simulink library "drv_ld_time_v0"  (R2016a)
settings: Solver=ode45  StartTime=0.0  StopTime=10.0  RelTol=1e-3
undefined symbols (not defined in the file): DiscIntNeverNeededParam, sMP
libraries: simulink x5
settings Model: Creator=LAUEREL  LastModifiedBy=UWLELKE
settings DataIOCC: LimitDataPoints=on  SaveFormat=Array
settings OptimizationCC: ExpressionDepthLimit=2147483647
settings DebuggingCC: UnderspecifiedInitializationDetection=Classic  MergeDetectMultiDrivingBlocksExec=none  SolverPrmCheckMsg=warning  StateNameClashWarn=warning
settings HardwareCC: ProdBitPerPointer=32  ProdLargestAtomicFloat=None  ProdIntDivRoundTo=Undefined  ProdEndianess=Unspecified  ProdWordSize=32  ProdHWDeviceType=32-bit Generic
settings ModelReferenceCC: PropagateSignalLabelsOutOfModel=off

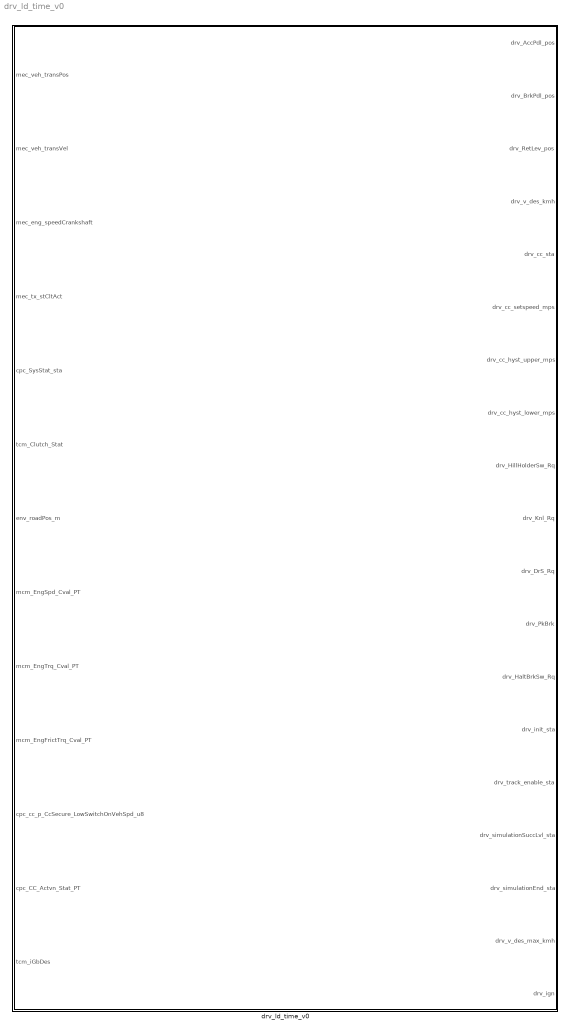
== system drv_ld_time_v0 ==
  drv_ld_time_v0 : Subsystem  TreatAsAtomicUnit=on  mask(DrivereDrive){aeroCdA_m2=sMP.human.drv.aeroCdA_m2, aeroRhoAirDensity_kgpm3=sMP.human.drv.aeroRhoAirDensity_kgpm3, coefReRollgVeh=sMP.human.drv.coefReRollgVeh, aGrv=sMP.human.drv.aGrv, Vehicle_Mass=sMP.human.drv.mass_gcw_kg, rdyn=sMP.human.drv.rdyn, CYC=sMP.bdry.env.CYC, gearration=sMP.human.drv.gearration, Ki_Accln=sMP.human.drv.Ki_Accln, Ki_breaking=sMP.human.drv.Ki_breaking, Veh_Speed_Breaking=sMP.human.drv.Veh_Speed_Breaking, veh_speed_accln=sMP.human.drv.veh_speed_accln, Kp_grad_Accln=sMP.human.drv.Kp_grad_Accln, Kp_grad_breaking=sMP.human.drv.Kp_grad_breaking, Grad_breaking=sMP.human.drv.Grad_breaking, Grad_Accln=sMP.human.drv.Grad_Accln, Mmax_motor=sMP.human.drv.Mmax_motor, vehPara_AccPdlCurve=sMP.human.drv.vehPara.AccPdlCurve, vehPara_BrkPdlCurve=sMP.human.drv.vehPara.BrkPdlCurve, Corr_const=sMP.human.drv.Corr_const, Kp_corr=sMP.human.drv.Kp_corr, Kp_acc_const=sMP.human.drv.Kp_acc_const, Kp_brk_const=sMP.human.drv.Kp_brk_const, corr_tuning=sMP.human.drv.corr_tuning, Ki_acc_const=sMP.human.drv.Ki_acc_const, Ki_brk_const=sMP.human.drv.Ki_brk_const, Kp_v=sMP.human.drv.Kp_v, Kp_acc=sMP.human.drv.Kp_acc, Kp_brk=sMP.human.drv.Kp_brk, Ki=sMP.human.drv.Ki, Ki_gain=sMP.human.drv.Ki_gain, refMass=sMP.human.drv.refMass}
      mask prompts: Vehicle_Mass "mass_gcw_kg"; CYC "cycleparameter"; gearration "gear ratio"
      mask help:
      | Set the struct variables for driver parameters (veh) and route data (cyc).
      |
      | eDrive Driver
      | This driver is able to drive time based cycles.

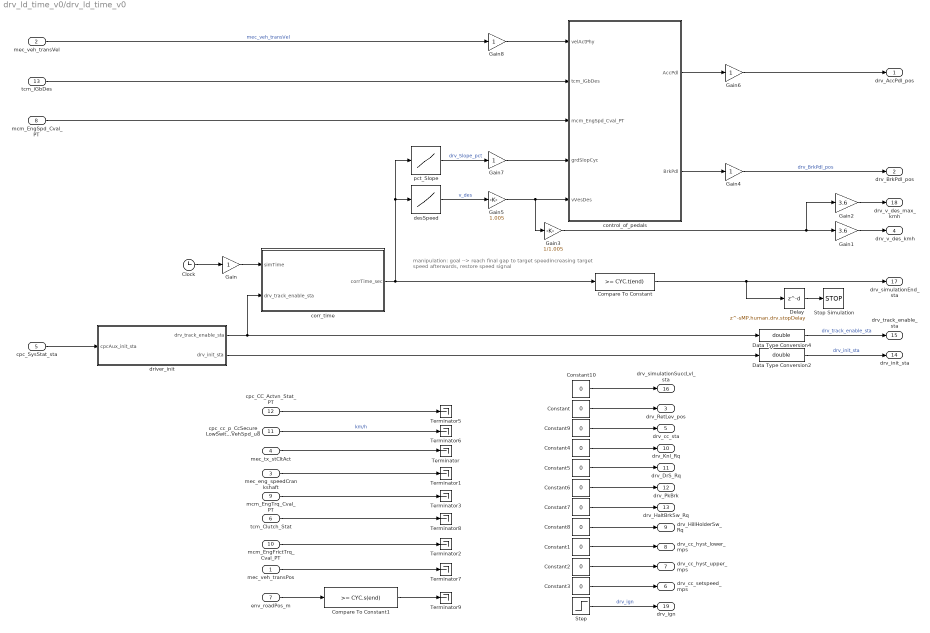
== system drv_ld_time_v0/drv_ld_time_v0 ==
  note: manipulation:
      | goal --> reach final gap to target speedincreasing target speed
      | afterwards, restore speed signal
  mec_veh_transPos : Inport
  mec_veh_transVel : Inport  Port=2
  mec_eng_speedCrankshaft : Inport  Port=3
  mec_tx_stCltAct : Inport  Port=4
  cpc_SysStat_sta : Inport  Port=5
  tcm_Clutch_Stat : Inport  Port=6
  env_roadPos_m : Inport  Port=7
  mcm_EngSpd_Cval_PT : Inport  Port=8
  mcm_EngTrq_Cval_PT : Inport  Port=9
  mcm_EngFrictTrq_Cval_PT : Inport  Port=10
  cpc_cc_p_CcSecure_LowSwitchOnVehSpd_u8 : Inport  Port=11
  cpc_CC_Actvn_Stat_PT : Inport  Port=12
  tcm_iGbDes : Inport  Port=13
  Clock : Clock
  Compare To Constant : simulink/Logic and Bit Operations/Compare To Constant  relop=>=  const=CYC.t(end)  OutDataTypeStr=boolean
  Compare To Constant1 : simulink/Logic and Bit Operations/Compare To Constant  relop=>=  const=CYC.s(end)  OutDataTypeStr=boolean
  Constant{,1..10} (11 alike) : Constant  Value=0
  Data Type Conversion2 : DataTypeConversion  OutDataTypeStr=double
  Data Type Conversion4 : DataTypeConversion  OutDataTypeStr=double
  Delay : Delay  DelayLength=sMP.human.drv.stopDelay  InitialCondition=0
  Gain : Gain  SampleTime=K
      mask init:
      | K = str2num(get_param(bdroot,'FixedStep'));
  Gain1 : Gain  Gain=3.6
  Gain2 : Gain  Gain=3.6
  Gain3 : Gain  Gain=1/1.005
      settings: AttributesFormatString=%<Gain>
  Gain{4,6..8} (4 alike) : Gain
  Gain5 : Gain  Gain=1.005
      settings: AttributesFormatString=%<Gain>
  Step : Step  Time=0.1  SampleTime=0
      settings: AttributesFormatString=%<Before> >> %<After> after %<Time>s
  Stop Simulation : Stop
  Terminator{,1..3,5..9} (9 alike) : Terminator
  control_of_pedals : Subsystem
  corr_time : Subsystem
  desSpeed : Lookup  InputValues=CYC.t  Table=CYC.v
  driver_init : Subsystem
  pct_Slope : Lookup  InputValues=CYC.t  Table=CYC.grade
  drv_AccPdl_pos : Outport
  drv_BrkPdl_pos : Outport  Port=2
  drv_RetLev_pos : Outport  Port=3
  drv_v_des_kmh : Outport  Port=4
  drv_cc_sta : Outport  Port=5
  drv_cc_setspeed_mps : Outport  Port=6
  drv_cc_hyst_upper_mps : Outport  Port=7
  drv_cc_hyst_lower_mps : Outport  Port=8
  drv_HillHolderSw_Rq : Outport  Port=9
  drv_Knl_Rq : Outport  Port=10
  drv_DrS_Rq : Outport  Port=11
  drv_PkBrk : Outport  Port=12
  drv_HaltBrkSw_Rq : Outport  Port=13
  drv_init_sta : Outport  Port=14
  drv_track_enable_sta : Outport  Port=15
  drv_simulationSuccLvl_sta : Outport  Port=16
  drv_simulationEnd_sta : Outport  Port=17
  drv_v_des_max_kmh : Outport  Port=18
  drv_ign : Outport  Port=19
  wires:
  mcm_EngFrictTrq_Cval_PT/1 -> Terminator2/1
  Constant10/1 -> drv_simulationSuccLvl_sta/1
  Delay/1 -> Stop Simulation/1
  Step/1 -> drv_ign/1  "drv_ign"
  tcm_iGbDes/1 -> control_of_pedals/2(tcm_iGbDes)
  mec_veh_transPos/1 -> Terminator7/1
  corr_time/1(corrTime_sec) -> pct_Slope/1, desSpeed/1, Compare To Constant/1
  Clock/1 -> Gain/1
  desSpeed/1 -> Gain5/1  "v_des"
  Constant/1 -> drv_RetLev_pos/1
  Constant9/1 -> drv_cc_sta/1
  Constant5/1 -> drv_DrS_Rq/1
  Constant6/1 -> drv_PkBrk/1
  Constant7/1 -> drv_HaltBrkSw_Rq/1
  Constant8/1 -> drv_HillHolderSw_Rq/1
  Constant4/1 -> drv_Knl_Rq/1
  Constant3/1 -> drv_cc_setspeed_mps/1
  Constant2/1 -> drv_cc_hyst_upper_mps/1
  Constant1/1 -> drv_cc_hyst_lower_mps/1
  tcm_Clutch_Stat/1 -> Terminator8/1
  mcm_EngTrq_Cval_PT/1 -> Terminator3/1
  mcm_EngSpd_Cval_PT/1 -> control_of_pedals/3(mcm_EngSpd_Cval_PT)
  mec_eng_speedCrankshaft/1 -> Terminator1/1
  mec_tx_stCltAct/1 -> Terminator/1
  cpc_cc_p_CcSecure_LowSwitchOnVehSpd_u8/1 -> Terminator6/1  "km/h"
  cpc_CC_Actvn_Stat_PT/1 -> Terminator5/1
  mec_veh_transVel/1 -> Gain8/1  "mec_veh_transVel"
  pct_Slope/1 -> Gain7/1  "drv_Slope_pct"
  cpc_SysStat_sta/1 -> driver_init/1(cpcAux_init_sta)
  driver_init/1(drv_track_enable_sta) -> corr_time/2(drv_track_enable_sta), Data Type Conversion4/1
  env_roadPos_m/1 -> Compare To Constant1/1
  Data Type Conversion4/1 -> drv_track_enable_sta/1  "drv_track_enable_sta"
  Data Type Conversion2/1 -> drv_init_sta/1  "drv_init_sta"
  driver_init/2(drv_init_sta) -> Data Type Conversion2/1
  Gain1/1 -> drv_v_des_kmh/1
  Gain2/1 -> drv_v_des_max_kmh/1
  Gain/1 -> corr_time/1(simTime)
  Compare To Constant/1 -> drv_simulationEnd_sta/1, Delay/1
  Compare To Constant1/1 -> Terminator9/1
  control_of_pedals/1(AccPdl) -> Gain6/1
  Gain4/1 -> drv_BrkPdl_pos/1  "drv_BrkPdl_pos"
  control_of_pedals/2(BrkPdl) -> Gain4/1
  Gain6/1 -> drv_AccPdl_pos/1
  Gain7/1 -> control_of_pedals/4(grdSlopCyc)
  Gain8/1 -> control_of_pedals/1(velActPhy)
  Gain3/1 -> Gain2/1, Gain1/1
  Gain5/1 -> Gain3/1, control_of_pedals/5(vVesDes)

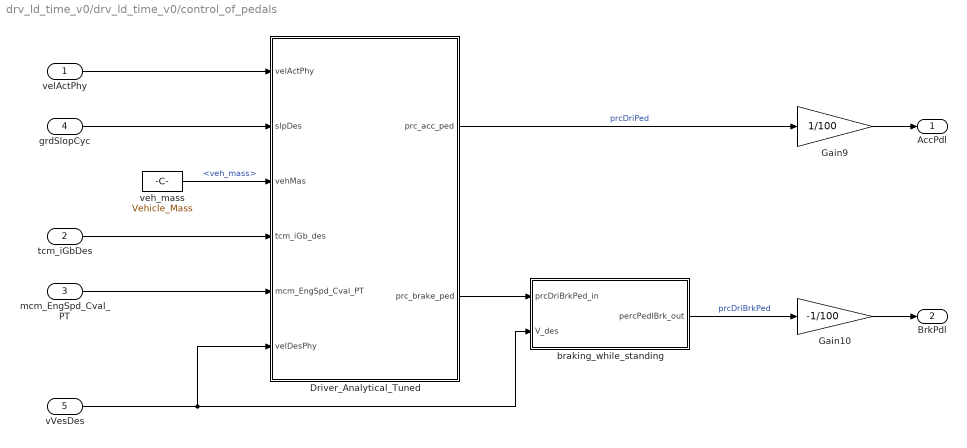
== system drv_ld_time_v0/drv_ld_time_v0/control_of_pedals ==
  velActPhy : Inport
  tcm_iGbDes : Inport  Port=2
  mcm_EngSpd_Cval_PT : Inport  Port=3
  grdSlopCyc : Inport  Port=4
  vVesDes : Inport  Port=5
  Driver_Analytical_Tuned : Subsystem
  Gain10 : Gain  Gain=-1/100
  Gain9 : Gain  Gain=1/100
  braking_while_standing : Subsystem
  veh_mass : Constant  Value=Vehicle_Mass
  AccPdl : Outport
  BrkPdl : Outport  Port=2
  wires:
  mcm_EngSpd_Cval_PT/1 -> Driver_Analytical_Tuned/5(mcm_EngSpd_Cval_PT)
  Driver_Analytical_Tuned/2(prc_brake_ped) -> braking_while_standing/1(prcDriBrkPed_in)
  braking_while_standing/1(percPedlBrk_out) -> Gain10/1  "prcDriBrkPed"
  tcm_iGbDes/1 -> Driver_Analytical_Tuned/4(tcm_iGb_des)
  veh_mass/1 -> Driver_Analytical_Tuned/3(vehMas)  "<veh_mass>"
  velActPhy/1 -> Driver_Analytical_Tuned/1(velActPhy)
  grdSlopCyc/1 -> Driver_Analytical_Tuned/2(slpDes)
  vVesDes/1 -> Driver_Analytical_Tuned/6(velDesPhy), braking_while_standing/2(V_des)
  Driver_Analytical_Tuned/1(prc_acc_ped) -> Gain9/1  "prcDriPed"
  Gain9/1 -> AccPdl/1
  Gain10/1 -> BrkPdl/1

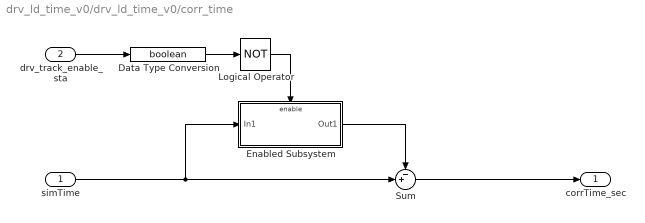
== system drv_ld_time_v0/drv_ld_time_v0/corr_time ==
  simTime : Inport
  drv_track_enable_sta : Inport  Port=2
  Data Type Conversion : DataTypeConversion  OutDataTypeStr=boolean
  Enabled Subsystem : Subsystem  TreatAsAtomicUnit=on
  Logical Operator : Logic  Operator=NOT  AllPortsSameDT=off  OutDataTypeStr=boolean
  Sum : Sum  Inputs=-+|
  corrTime_sec : Outport
  wires:
  Data Type Conversion/1 -> Logical Operator/1
  Sum/1 -> corrTime_sec/1
  Enabled Subsystem/1(Out1) -> Sum/1
  Logical Operator/1 -> Enabled Subsystem/Enable
  drv_track_enable_sta/1 -> Data Type Conversion/1
  simTime/1 -> Sum/2, Enabled Subsystem/1(In1)

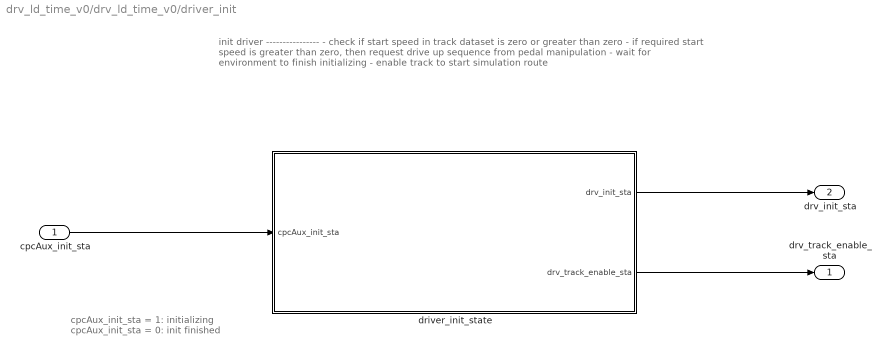
== system drv_ld_time_v0/drv_ld_time_v0/driver_init ==
  note: init driver
      | ----------------
      | - check if start speed in track dataset is zero or greater than zero
      | - if required start speed is greater than zero, then request drive up sequence from pedal manipulation
      | - wait for environment to finish initializing
      | - enable track to start simulation route
  note: cpcAux_init_sta = 1: initializing
      | cpcAux_init_sta = 0: init finished
  cpcAux_init_sta : Inport
  driver_init_state : Stateflow chart  TreatAsAtomicUnit=on
  drv_track_enable_sta : Outport
  drv_init_sta : Outport  Port=2
  wires:
  driver_init_state/1(drv_init_sta) -> drv_init_sta/1
  driver_init_state/2(drv_track_enable_sta) -> drv_track_enable_sta/1
  cpcAux_init_sta/1 -> driver_init_state/1(cpcAux_init_sta)

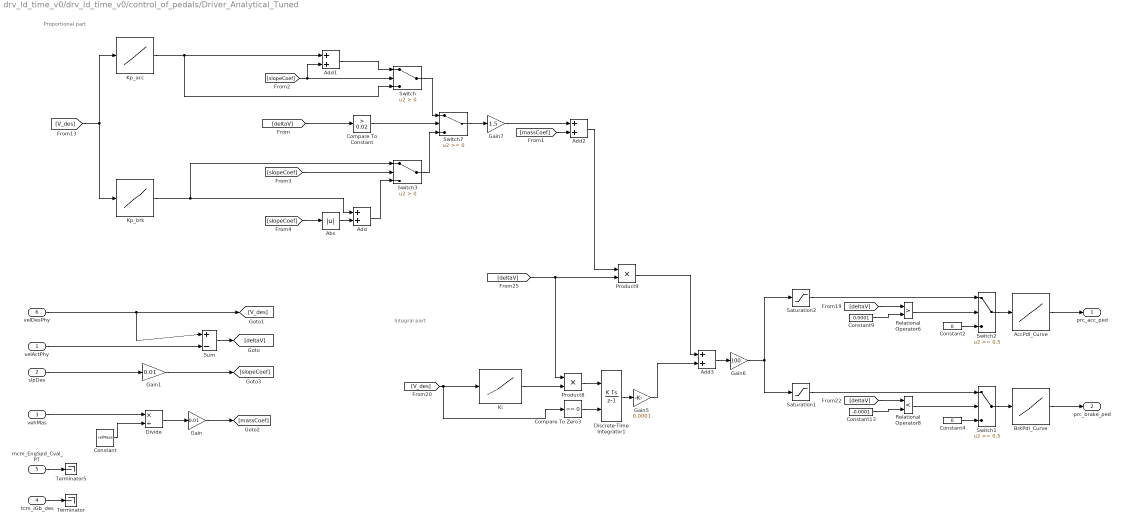
== system drv_ld_time_v0/drv_ld_time_v0/control_of_pedals/Driver_Analytical_Tuned ==
  note: Integral part
  note: Proportional part
  velActPhy : Inport
  slpDes : Inport  Port=2
  vehMas : Inport  Port=3
  tcm_iGb_des : Inport  Port=4
  mcm_EngSpd_Cval_PT : Inport  Port=5
  velDesPhy : Inport  Port=6
  Abs : Abs
  AccPdl_Curve : Lookup_n-D  NumberOfTableDimensions=1  BreakpointsForDimension1=vehPara_AccPdlCurve(:,1)  Table=vehPara_AccPdlCurve(:,2)  InternalRulePriority=Speed  RndMeth=Simplest  InputSameDT=on
  Add{,1..3} (4 alike) : Sum
  BrkPdl_Curve : Lookup_n-D  NumberOfTableDimensions=1  BreakpointsForDimension1=vehPara_BrkPdlCurve(:,1)  Table=vehPara_BrkPdlCurve(:,2)  InternalRulePriority=Speed  RndMeth=Simplest  InputSameDT=on
  Compare To Constant : simulink/Logic and Bit Operations/Compare To Constant  relop=>  const=0.02  OutDataTypeStr=boolean
  Compare To Zero3 : simulink/Logic and Bit Operations/Compare To Zero  relop===  OutDataTypeStr=boolean
  Constant : Constant  Value=refMass
      settings: AttributesFormatString=%<Value>
  Constant13 : Constant  Value=-0.0001
  Constant2 : Constant  Value=0
  Constant4 : Constant  Value=0
  Constant9 : Constant  Value=0.0001
  Discrete-Time Integrator1 : DiscreteIntegrator  ExternalReset=level  SampleTime=-1  LimitOutput=on  UpperSaturationLimit=7500  LowerSaturationLimit=-7500  ICPrevOutput=DiscIntNeverNeededParam  ICPrevScaledInput=DiscIntNeverNeededParam
  Divide : Product  Inputs=*/
  Gain : Gain  Gain=0.01
      settings: AttributesFormatString=%<Gain>
  Gain1 : Gain  Gain=0.01
  Gain5 : Gain  Gain=0.0001
      settings: AttributesFormatString=%<Gain>
  Gain6 : Gain  Gain=100
  Gain7 : Gain  Gain=1.5
      settings: AttributesFormatString=%<Gain>
  Ki : Lookup_n-D  NumberOfTableDimensions=1  BreakpointsForDimension1=[0,10,20,30,40,50,60,70,80]  BreakpointsForDimension2=Veh_Speed_Breaking  Table=[0.01,0.015,0.02,0.0225,0.03,0.035,0.04,0.045,0.05]  RndMeth=Simplest  InputSameDT=on
  Kp_acc : Lookup_n-D  NumberOfTableDimensions=1  BreakpointsForDimension1=Kp_acc(2,:)  BreakpointsForDimension2=Veh_Speed_Breaking  Table=Kp_acc(1,:)  RndMeth=Simplest  InputSameDT=on
  Kp_brk : Lookup_n-D  NumberOfTableDimensions=1  BreakpointsForDimension1=[0,10,20,30,40,50,60,70,80,90,100]  BreakpointsForDimension2=Veh_Speed_Breaking  Table=[1,1.25,1.25,1.5,1.5,1.5,1.7,1.8,1.8,1.8,2]*0.1  RndMeth=Simplest  InputSameDT=on
  Product8 : Product
  Product9 : Product
  Relational Operator6 : RelationalOperator  Operator=>  OutDataTypeStr=uint(8)
  Relational Operator8 : RelationalOperator  Operator=<  OutDataTypeStr=uint(8)
  Saturation1 : Saturate  UpperLimit=0  LowerLimit=-100
      settings: AttributesFormatString=%<UpperLimit>\n%<LowerLimit>
  Saturation2 : Saturate  UpperLimit=100  LowerLimit=0
      settings: AttributesFormatString=%<UpperLimit>\n%<LowerLimit>
  Sum : Sum  Inputs=|+-
  Switch : Switch  Criteria=u2 > Threshold
  Switch1 : Switch  Threshold=0.5
  Switch2 : Switch  Threshold=0.5
  Switch3 : Switch  Criteria=u2 > Threshold
  Switch7 : Switch
  Terminator : Terminator
  Terminator5 : Terminator
  prc_acc_ped : Outport
  prc_brake_ped : Outport  Port=2
  wires:
  Gain7/1 -> Add2/1
  Gain/1 -> [massCoef]
  Gain1/1 -> [slopeCoef]
  [massCoef] -> Add2/2
  Divide/1 -> Gain/1
  Add2/1 -> Product9/1
  Switch7/1 -> Gain7/1
  [deltaV] -> Product8/1, Product9/2
  Add1/1 -> Switch/1
  Product9/1 -> Add3/1
  Kp_brk/1 -> Switch3/1, Add/1
  Switch3/1 -> Switch7/3
  [slopeCoef] -> Switch3/2
  Kp_acc/1 -> Switch/3, Add1/1
  Switch/1 -> Switch7/1
  Constant/1 -> Divide/2
  Sum/1 -> [deltaV]
  Compare To Constant/1 -> Switch7/2
  Discrete-Time Integrator1/1 -> Gain5/1
  Compare To Zero3/1 -> Discrete-Time Integrator1/2
  [V_des] -> Ki/1, Compare To Zero3/1
  [deltaV] -> Compare To Constant/1
  [V_des] -> Kp_acc/1, Kp_brk/1
  Gain6/1 -> Saturation1/1, Saturation2/1
  Add3/1 -> Gain6/1
  Product8/1 -> Discrete-Time Integrator1/1
  Relational Operator8/1 -> Switch1/2
  [deltaV] -> Relational Operator8/1
  Constant13/1 -> Relational Operator8/2
  Relational Operator6/1 -> Switch2/2
  [deltaV] -> Relational Operator6/1
  Constant9/1 -> Relational Operator6/2
  mcm_EngSpd_Cval_PT/1 -> Terminator5/1
  velActPhy/1 -> Sum/2
  AccPdl_Curve/1 -> prc_acc_ped/1
  BrkPdl_Curve/1 -> prc_brake_ped/1
  tcm_iGb_des/1 -> Terminator/1
  velDesPhy/1 -> [V_des], Sum/1
  slpDes/1 -> Gain1/1
  vehMas/1 -> Divide/1
  Saturation2/1 -> Switch2/1
  Saturation1/1 -> Switch1/1
  Switch2/1 -> AccPdl_Curve/1
  Switch1/1 -> BrkPdl_Curve/1
  Constant4/1 -> Switch1/3
  Constant2/1 -> Switch2/3
  [slopeCoef] -> Switch/2, Add1/2
  [slopeCoef] -> Abs/1
  Abs/1 -> Add/2
  Add/1 -> Switch3/3
  Gain5/1 -> Add3/2
  Ki/1 -> Product8/2

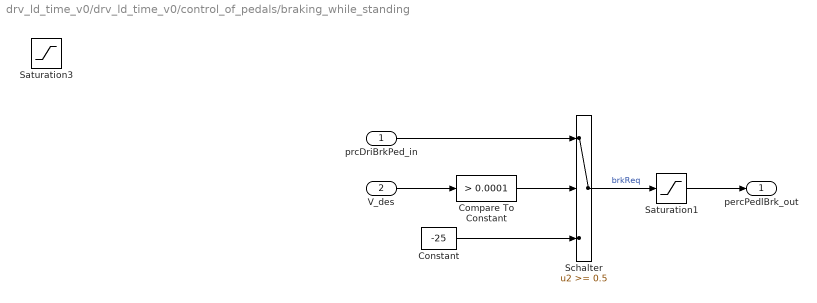
== system drv_ld_time_v0/drv_ld_time_v0/control_of_pedals/braking_while_standing ==
  prcDriBrkPed_in : Inport
  V_des : Inport  Port=2
  Compare To Constant : simulink/Logic and Bit Operations/Compare To Constant  relop=>  const=0.0001  OutDataTypeStr=boolean
  Constant : Constant  Value=-25
      settings: AttributesFormatString=%<Value>
  Saturation1 : Saturate  UpperLimit=0  LowerLimit=-100
      settings: AttributesFormatString=%<UpperLimit>\n%<LowerLimit>
  Saturation3 : Saturate  UpperLimit=0  LowerLimit=-100
      settings: AttributesFormatString=%<UpperLimit>\n%<LowerLimit>
  Schalter : Switch  Threshold=0.5  SaturateOnIntegerOverflow=on
      settings: AttributesFormatString=%<Criteria>(%<Threshold>)
  percPedlBrk_out : Outport  Description=[%]
      settings: AttributesFormatString=%<Description>
  wires:
  Schalter/1 -> Saturation1/1  "brkReq"
  Constant/1 -> Schalter/3
  prcDriBrkPed_in/1 -> Schalter/1
  V_des/1 -> Compare To Constant/1
  Compare To Constant/1 -> Schalter/2
  Saturation1/1 -> percPedlBrk_out/1

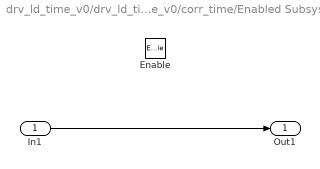
== system drv_ld_time_v0/drv_ld_time_v0/corr_time/Enabled Subsystem ==
  In1 : Inport
  Enable : EnablePort
  Out1 : Outport
  wires:
  In1/1 -> Out1/1

== stateflow chart drv_ld_time_v0/driver_init/driver_init_state ==
  settings: enableNonTerminalStates=1
  note: vehPara_type:
      | 1: teachIn procedure
      | 0: w/o teachIn
      |
      | tbd
  state Init
    en:
    drv_init_sta = 0;
    drv_track_enable_sta = 0;
  state Final
    en:
    drv_init_sta = 1;
    drv_track_enable_sta = 1;
    du:
  (default) -> Init
  Init -> Final : [cpcAux_init_sta == 0]
  data: cpcAux_init_sta input; drv_init_sta output double; drv_track_enable_sta output double; count local double
